simulink model "sim3"  (R2015b)
settings: Solver=VariableStepAuto  StartTime=0.0  StopTime=10.0  RelTol=1e-3
settings Model: Creator=z  LastModifiedBy=z

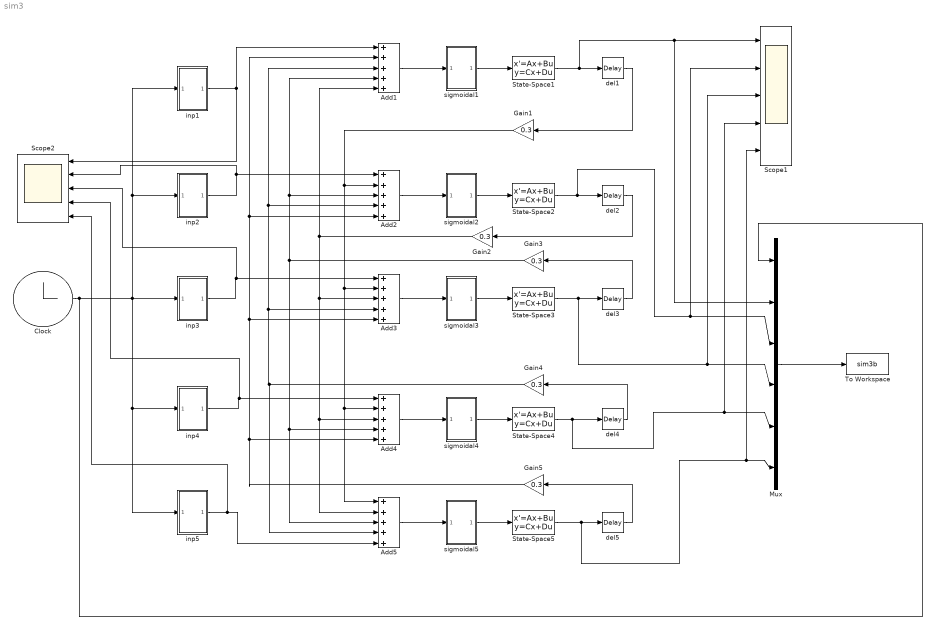
== system sim3 ==
  Add{1..5} (5 alike) : Sum  Inputs=+++++
  Clock : Clock
  Gain{1..5} (5 alike) : Gain  Gain=0.3
  Mux : Mux  Inputs=6
  Scope1 : Scope  NumInputPorts=5
  Scope2 : Scope  NumInputPorts=5
  State-Space{1..5} (5 alike) : StateSpace  A=-50  B=50  D=0  X0=.5  ContinuousStateAttributes='x'
  To Workspace : ToWorkspace  VariableName=sim3b  SampleTime=-1
  del{1..5} (5 alike) : TransportDelay  DelayTime=2  InitialOutput=.5
  inp1 : Subsystem
  inp2 : Subsystem
  inp3 : Subsystem
  inp4 : Subsystem
  inp5 : Subsystem
  sigmoidal1 : Subsystem
  sigmoidal2 : Subsystem
  sigmoidal3 : Subsystem
  sigmoidal4 : Subsystem
  sigmoidal5 : Subsystem
  wires:
  Mux/1 -> To Workspace/1
  Clock/1 -> Mux/1, inp3/1(In1), inp2/1(In1), inp1/1(In1), inp4/1(In1), inp5/1(In1)
  Add1/1 -> sigmoidal1/1(In1)
  State-Space1/1 -> Mux/2, Scope1/1, del1/1
  sigmoidal1/1(Out1) -> State-Space1/1
  Add3/1 -> sigmoidal3/1(In1)
  State-Space3/1 -> Mux/4, Scope1/3, del3/1
  sigmoidal3/1(Out1) -> State-Space3/1
  Add4/1 -> sigmoidal4/1(In1)
  sigmoidal4/1(Out1) -> State-Space4/1
  Add2/1 -> sigmoidal2/1(In1)
  State-Space2/1 -> Mux/3, Scope1/2, del2/1
  sigmoidal2/1(Out1) -> State-Space2/1
  Add5/1 -> sigmoidal5/1(In1)
  State-Space5/1 -> Mux/6, Scope1/5, del5/1
  sigmoidal5/1(Out1) -> State-Space5/1
  inp1/1(Out1) -> Scope2/1, Add1/1
  inp2/1(Out1) -> Add2/1, Scope2/2
  inp3/1(Out1) -> Scope2/3, Add3/1
  inp4/1(Out1) -> Scope2/4, Add4/1
  inp5/1(Out1) -> Scope2/5, Add5/5
  del5/1 -> Gain5/1
  del4/1 -> Gain4/1
  del3/1 -> Gain3/1
  del2/1 -> Gain2/1
  del1/1 -> Gain1/1
  State-Space4/1 -> Mux/5, Scope1/4, del4/1
  Gain5/1 -> Add4/5, Add3/5, Add2/5, Add1/2
  Gain4/1 -> Add3/4, Add2/4, Add1/3, Add5/4
  Gain3/1 -> Add5/3, Add4/4, Add2/3, Add1/4
  Gain2/1 -> Add3/3, Add5/2, Add4/3, Add1/5
  Gain1/1 -> Add2/2, Add3/2, Add4/2, Add5/1

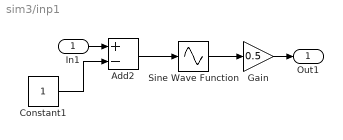
== system sim3/inp1 ==
  In1 : Inport
  Add2 : Sum  Inputs=+-
  Constant1 : Constant
  Gain : Gain  Gain=0.5
  Sine Wave Function : Sin  TimeSource=Use external signal  SampleTime=0
  Out1 : Outport
  wires:
  In1/1 -> Add2/1
  Gain/1 -> Out1/1
  Sine Wave Function/1 -> Gain/1
  Add2/1 -> Sine Wave Function/1
  Constant1/1 -> Add2/2

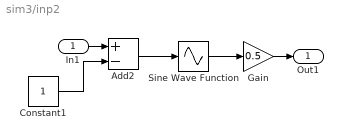
== system sim3/inp2 ==
  In1 : Inport
  Add2 : Sum  Inputs=+-
  Constant1 : Constant
  Gain : Gain  Gain=0.5
  Sine Wave Function : Sin  TimeSource=Use external signal  Frequency=2  SampleTime=0
  Out1 : Outport
  wires:
  In1/1 -> Add2/1
  Gain/1 -> Out1/1
  Sine Wave Function/1 -> Gain/1
  Add2/1 -> Sine Wave Function/1
  Constant1/1 -> Add2/2

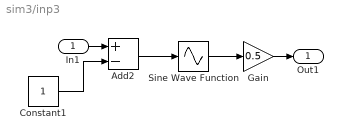
== system sim3/inp3 ==
  In1 : Inport
  Add2 : Sum  Inputs=+-
  Constant1 : Constant
  Gain : Gain  Gain=0.5
  Sine Wave Function : Sin  TimeSource=Use external signal  Frequency=3  SampleTime=0
  Out1 : Outport
  wires:
  In1/1 -> Add2/1
  Gain/1 -> Out1/1
  Sine Wave Function/1 -> Gain/1
  Add2/1 -> Sine Wave Function/1
  Constant1/1 -> Add2/2

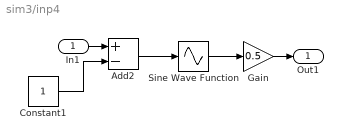
== system sim3/inp4 ==
  In1 : Inport
  Add2 : Sum  Inputs=+-
  Constant1 : Constant
  Gain : Gain  Gain=0.5
  Sine Wave Function : Sin  TimeSource=Use external signal  Frequency=4  SampleTime=0
  Out1 : Outport
  wires:
  In1/1 -> Add2/1
  Gain/1 -> Out1/1
  Sine Wave Function/1 -> Gain/1
  Add2/1 -> Sine Wave Function/1
  Constant1/1 -> Add2/2

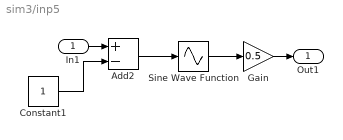
== system sim3/inp5 ==
  In1 : Inport
  Add2 : Sum  Inputs=+-
  Constant1 : Constant
  Gain : Gain  Gain=0.5
  Sine Wave Function : Sin  TimeSource=Use external signal  Frequency=5  SampleTime=0
  Out1 : Outport
  wires:
  In1/1 -> Add2/1
  Gain/1 -> Out1/1
  Sine Wave Function/1 -> Gain/1
  Add2/1 -> Sine Wave Function/1
  Constant1/1 -> Add2/2

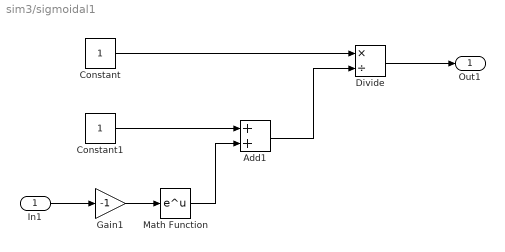
== system sim3/sigmoidal1 ==
  In1 : Inport
  Add1 : Sum
  Constant : Constant
  Constant1 : Constant
  Divide : Product  Inputs=*/
  Gain1 : Gain  Gain=-1
  Math Function : Math  SaturateOnIntegerOverflow=on
  Out1 : Outport
  wires:
  Constant1/1 -> Add1/1
  Gain1/1 -> Math Function/1
  Divide/1 -> Out1/1
  Constant/1 -> Divide/1
  In1/1 -> Gain1/1
  Add1/1 -> Divide/2
  Math Function/1 -> Add1/2

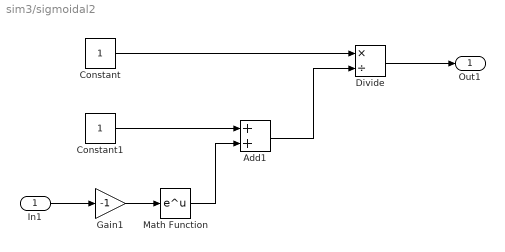
== system sim3/sigmoidal2 ==
  In1 : Inport
  Add1 : Sum
  Constant : Constant
  Constant1 : Constant
  Divide : Product  Inputs=*/
  Gain1 : Gain  Gain=-1
  Math Function : Math  SaturateOnIntegerOverflow=on
  Out1 : Outport
  wires:
  Constant1/1 -> Add1/1
  Gain1/1 -> Math Function/1
  Divide/1 -> Out1/1
  Constant/1 -> Divide/1
  In1/1 -> Gain1/1
  Add1/1 -> Divide/2
  Math Function/1 -> Add1/2

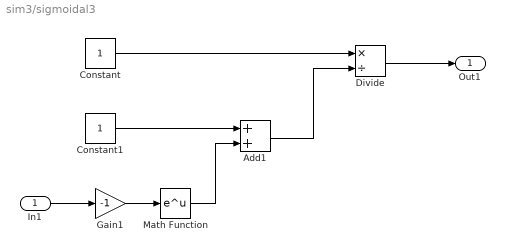
== system sim3/sigmoidal3 ==
  In1 : Inport
  Add1 : Sum
  Constant : Constant
  Constant1 : Constant
  Divide : Product  Inputs=*/
  Gain1 : Gain  Gain=-1
  Math Function : Math  SaturateOnIntegerOverflow=on
  Out1 : Outport
  wires:
  Constant1/1 -> Add1/1
  Gain1/1 -> Math Function/1
  Divide/1 -> Out1/1
  Constant/1 -> Divide/1
  In1/1 -> Gain1/1
  Add1/1 -> Divide/2
  Math Function/1 -> Add1/2

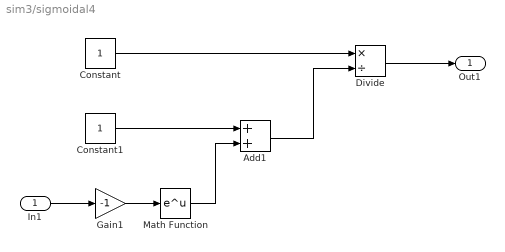
== system sim3/sigmoidal4 ==
  In1 : Inport
  Add1 : Sum
  Constant : Constant
  Constant1 : Constant
  Divide : Product  Inputs=*/
  Gain1 : Gain  Gain=-1
  Math Function : Math  SaturateOnIntegerOverflow=on
  Out1 : Outport
  wires:
  Constant1/1 -> Add1/1
  Gain1/1 -> Math Function/1
  Divide/1 -> Out1/1
  Constant/1 -> Divide/1
  In1/1 -> Gain1/1
  Add1/1 -> Divide/2
  Math Function/1 -> Add1/2

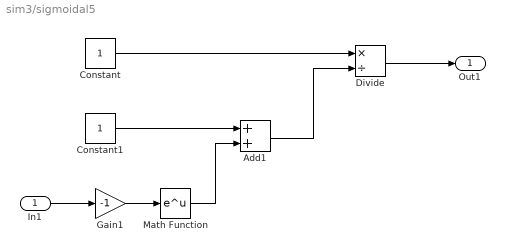
== system sim3/sigmoidal5 ==
  In1 : Inport
  Add1 : Sum
  Constant : Constant
  Constant1 : Constant
  Divide : Product  Inputs=*/
  Gain1 : Gain  Gain=-1
  Math Function : Math  SaturateOnIntegerOverflow=on
  Out1 : Outport
  wires:
  Constant1/1 -> Add1/1
  Gain1/1 -> Math Function/1
  Divide/1 -> Out1/1
  Constant/1 -> Divide/1
  In1/1 -> Gain1/1
  Add1/1 -> Divide/2
  Math Function/1 -> Add1/2
